simulink model "LabIVquestaoum"  (Simulink 7.1)
settings: Solver=ode45  StartTime=0.0  StopTime=100  RelTol=1e-3
settings Model: Creator=ALUNO  LastModifiedBy=ALUNO

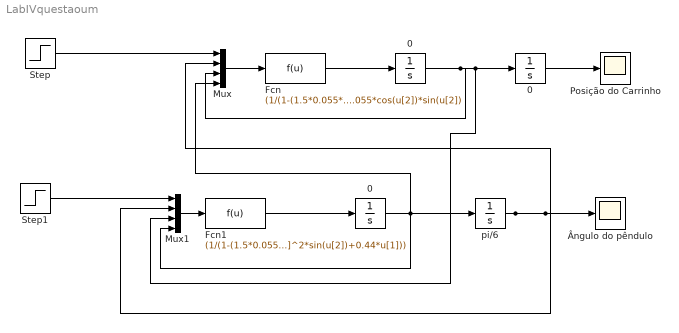
== system LabIVquestaoum ==
  0 : Integrator
  "0 " : Integrator
  "0  " : Integrator
  Fcn : Fcn  Expr=(1/(1-(1.5*0.055*(cos(u[2]))^2)))*(-0.22*u[3]+0.055*u[4]^2*sin(u[2]))+0.44*u[1]+14.71*0.055*cos(u[2])*sin(u[2])
  Fcn1 : Fcn  Expr=(1/(1-(1.5*0.055*(cos(u[2]))^2)))*(-14.71*sin(u[2])-1.5*cos(u[2])*(-0.22*u[3]+0.055*u[4]^2*sin(u[2])+0.44*u[1]))
  Mux : Mux
  Mux1 : Mux
  Posição do Carrinho : Scope
      settings: MaxDataPoints=100000
  Step : Step  Time=0  After=0  SampleTime=0
  Step1 : Step  Time=0  After=0  SampleTime=0
  pi/6 : Integrator  InitialCondition=pi/6
  Ângulo do pêndulo : Scope
      settings: MaxDataPoints=100000
  wires:
  Fcn/1 -> "0 "/1
  "0 "/1 -> Mux/3, 0/1, Mux1/3
  0/1 -> Posição do Carrinho/1
  Fcn1/1 -> "0  "/1
  "0  "/1 -> pi/6/1, Mux1/4, Mux/4
  pi/6/1 -> Ângulo do pêndulo/1, Mux/2, Mux1/2
  Mux/1 -> Fcn/1
  Mux1/1 -> Fcn1/1
  Step/1 -> Mux/1
  Step1/1 -> Mux1/1
